simulink model "kpt_simulink_library"  (R2016b)
settings: Solver=VariableStepAuto  StartTime=0.0  StopTime=10.0  RelTol=1e-3
settings Model: Creator=u18b15  LastModifiedBy=u18b15

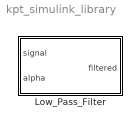
== system kpt_simulink_library ==
  Low_Pass_Filter : Subsystem

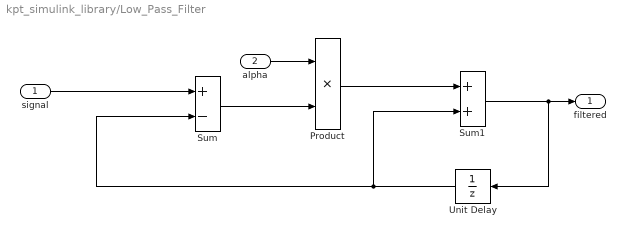
== system kpt_simulink_library/Low_Pass_Filter ==
  signal : Inport
  alpha : Inport  Port=2
  Product : Product
  Sum : Sum  Inputs=+-
  Sum1 : Sum
  Unit Delay : UnitDelay  SampleTime=-1
  filtered : Outport
  wires:
  alpha/1 -> Product/1
  signal/1 -> Sum/1
  Sum/1 -> Product/2
  Product/1 -> Sum1/1
  Sum1/1 -> Unit Delay/1, filtered/1
  Unit Delay/1 -> Sum/2, Sum1/2
